simulink model "ALL_JP360_DBW_V6_5_1103"  (R2022a)
settings: Solver=FixedStepAuto  StartTime=0.0  StopTime=inf  FixedStep=0.01  RelTol=1e-3  EnableMultiTasking=on
model workspace (MAT data in the model file):
  g = 9.8
undefined symbols (not defined in the file or in its folder): canChannel, delta_v_p, IPM_Line_C0, IPM_Line_C1, IPM_Line_C2, IPM_Line_C3, M, M_p, MRR_ObjDistX, MRR_ObjDistY, MRR_ObjFusionCamID, MRR_ObjFusionSig, MRR_ObjID, MRR_ObjRelVelX, MRR_ObjRelVelY, MRR_ObjType, MRR_ObjUpdFlg, none, obj_vaild, untracktime, V, videoinput
libraries: canfdmsglib x230, canfdlib x76, slpidlib x24, simulink x18, dspstat3 x14, ctrlSharedLib x1, simulink_extras x1, imaqlib x1, realtime_pacer_lib x1, dspvision x1, visionsinks x1
(part 6 of 55)

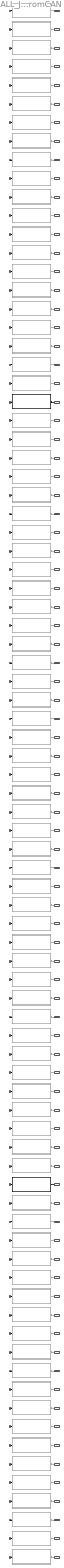
== system ALL_JP360_DBW_V6_5_1103/MsgFromCAN/SRR_ADCU_MsgFromCAN ==
  SRR_ADCU_FLR_AssistSysSt_0x71FromInData : Inport  OutDataTypeStr=Bus:CAN_FD_MESSAGE_BUS
  SRR_ADCU_FLR_Freespace_0x1E1FromInData : Inport  Port=2  OutDataTypeStr=Bus:CAN_FD_MESSAGE_BUS
  SRR_ADCU_FLR_Freespace_0x1E2FromInData : Inport  Port=3  OutDataTypeStr=Bus:CAN_FD_MESSAGE_BUS
  SRR_ADCU_FLR_Freespace_0x1E3FromInData : Inport  Port=4  OutDataTypeStr=Bus:CAN_FD_MESSAGE_BUS
  SRR_ADCU_FLR_Freespace_0x1E4FromInData : Inport  Port=5  OutDataTypeStr=Bus:CAN_FD_MESSAGE_BUS
  SRR_ADCU_FLR_OBJPos10_0x19AFromInData : Inport  Port=6  OutDataTypeStr=Bus:CAN_FD_MESSAGE_BUS
  SRR_ADCU_FLR_OBJPos11_0x19BFromInData : Inport  Port=7  OutDataTypeStr=Bus:CAN_FD_MESSAGE_BUS
  SRR_ADCU_FLR_OBJPos12_0x19CFromInData : Inport  Port=8  OutDataTypeStr=Bus:CAN_FD_MESSAGE_BUS
  SRR_ADCU_FLR_OBJPos13_0x19DFromInData : Inport  Port=9  OutDataTypeStr=Bus:CAN_FD_MESSAGE_BUS
  SRR_ADCU_FLR_OBJPos14_0x19EFromInData : Inport  Port=10  OutDataTypeStr=Bus:CAN_FD_MESSAGE_BUS
  SRR_ADCU_FLR_OBJPos15_0x1A1FromInData : Inport  Port=11  OutDataTypeStr=Bus:CAN_FD_MESSAGE_BUS
  SRR_ADCU_FLR_OBJPos16_0x1A2FromInData : Inport  Port=12  OutDataTypeStr=Bus:CAN_FD_MESSAGE_BUS
  SRR_ADCU_FLR_OBJPos1_0x191FromInData : Inport  Port=13  OutDataTypeStr=Bus:CAN_FD_MESSAGE_BUS
  SRR_ADCU_FLR_OBJPos2_0x192FromInData : Inport  Port=14  OutDataTypeStr=Bus:CAN_FD_MESSAGE_BUS
  SRR_ADCU_FLR_OBJPos3_0x193FromInData : Inport  Port=15  OutDataTypeStr=Bus:CAN_FD_MESSAGE_BUS
  SRR_ADCU_FLR_OBJPos4_0x194FromInData : Inport  Port=16  OutDataTypeStr=Bus:CAN_FD_MESSAGE_BUS
  SRR_ADCU_FLR_OBJPos5_0x195FromInData : Inport  Port=17  OutDataTypeStr=Bus:CAN_FD_MESSAGE_BUS
  SRR_ADCU_FLR_OBJPos6_0x196FromInData : Inport  Port=18  OutDataTypeStr=Bus:CAN_FD_MESSAGE_BUS
  SRR_ADCU_FLR_OBJPos7_0x197FromInData : Inport  Port=19  OutDataTypeStr=Bus:CAN_FD_MESSAGE_BUS
  SRR_ADCU_FLR_OBJPos8_0x198FromInData : Inport  Port=20  OutDataTypeStr=Bus:CAN_FD_MESSAGE_BUS
  SRR_ADCU_FLR_OBJPos9_0x199FromInData : Inport  Port=21  OutDataTypeStr=Bus:CAN_FD_MESSAGE_BUS
  SRR_ADCU_FRR_AssistSysSt_0x72FromInData : Inport  Port=22  OutDataTypeStr=Bus:CAN_FD_MESSAGE_BUS
  SRR_ADCU_FRR_Freespace_1E6FromInData : Inport  Port=23  OutDataTypeStr=Bus:CAN_FD_MESSAGE_BUS
  SRR_ADCU_FRR_Freespace_1E7FromInData : Inport  Port=24  OutDataTypeStr=Bus:CAN_FD_MESSAGE_BUS
  SRR_ADCU_FRR_Freespace_1E8FromInData : Inport  Port=25  OutDataTypeStr=Bus:CAN_FD_MESSAGE_BUS
  SRR_ADCU_FRR_Freespace_1E9FromInData : Inport  Port=26  OutDataTypeStr=Bus:CAN_FD_MESSAGE_BUS
  SRR_ADCU_FRR_OBJPos10_0x1ACFromInData : Inport  Port=27  OutDataTypeStr=Bus:CAN_FD_MESSAGE_BUS
  SRR_ADCU_FRR_OBJPos11_0x1ADFromInData : Inport  Port=28  OutDataTypeStr=Bus:CAN_FD_MESSAGE_BUS
  SRR_ADCU_FRR_OBJPos12_0x1AEFromInData : Inport  Port=29  OutDataTypeStr=Bus:CAN_FD_MESSAGE_BUS
  SRR_ADCU_FRR_OBJPos13_0x1B0FromInData : Inport  Port=30  OutDataTypeStr=Bus:CAN_FD_MESSAGE_BUS
  SRR_ADCU_FRR_OBJPos14_0x1B1FromInData : Inport  Port=31  OutDataTypeStr=Bus:CAN_FD_MESSAGE_BUS
  SRR_ADCU_FRR_OBJPos15_0x1B2FromInData : Inport  Port=32  OutDataTypeStr=Bus:CAN_FD_MESSAGE_BUS
  SRR_ADCU_FRR_OBJPos16_0x1B3FromInData : Inport  Port=33  OutDataTypeStr=Bus:CAN_FD_MESSAGE_BUS
  SRR_ADCU_FRR_OBJPos1_0x1A3FromInData : Inport  Port=34  OutDataTypeStr=Bus:CAN_FD_MESSAGE_BUS
  SRR_ADCU_FRR_OBJPos2_0x1A4FromInData : Inport  Port=35  OutDataTypeStr=Bus:CAN_FD_MESSAGE_BUS
  SRR_ADCU_FRR_OBJPos3_0x1A5FromInData : Inport  Port=36  OutDataTypeStr=Bus:CAN_FD_MESSAGE_BUS
  SRR_ADCU_FRR_OBJPos4_0x1A6FromInData : Inport  Port=37  OutDataTypeStr=Bus:CAN_FD_MESSAGE_BUS
  SRR_ADCU_FRR_OBJPos5_0x1A7FromInData : Inport  Port=38  OutDataTypeStr=Bus:CAN_FD_MESSAGE_BUS
  SRR_ADCU_FRR_OBJPos6_0x1A8FromInData : Inport  Port=39  OutDataTypeStr=Bus:CAN_FD_MESSAGE_BUS
  SRR_ADCU_FRR_OBJPos7_0x1A9FromInData : Inport  Port=40  OutDataTypeStr=Bus:CAN_FD_MESSAGE_BUS
  SRR_ADCU_FRR_OBJPos8_0x1AAFromInData : Inport  Port=41  OutDataTypeStr=Bus:CAN_FD_MESSAGE_BUS
  SRR_ADCU_FRR_OBJPos9_0x1ABFromInData : Inport  Port=42  OutDataTypeStr=Bus:CAN_FD_MESSAGE_BUS
  SRR_ADCU_RLR_AssistSysSt_0x74FromInData : Inport  Port=43  OutDataTypeStr=Bus:CAN_FD_MESSAGE_BUS
  SRR_ADCU_RLR_Freespace_0x1F1FromInData : Inport  Port=44  OutDataTypeStr=Bus:CAN_FD_MESSAGE_BUS
  SRR_ADCU_RLR_Freespace_0x1F2FromInData : Inport  Port=45  OutDataTypeStr=Bus:CAN_FD_MESSAGE_BUS
  SRR_ADCU_RLR_Freespace_0x1F3FromInData : Inport  Port=46  OutDataTypeStr=Bus:CAN_FD_MESSAGE_BUS
  SRR_ADCU_RLR_Freespace_0x1F4FromInData : Inport  Port=47  OutDataTypeStr=Bus:CAN_FD_MESSAGE_BUS
  SRR_ADCU_RLR_OBJPos10_0x1CDFromInData : Inport  Port=48  OutDataTypeStr=Bus:CAN_FD_MESSAGE_BUS
  SRR_ADCU_RLR_OBJPos11_0x1CEFromInData : Inport  Port=49  OutDataTypeStr=Bus:CAN_FD_MESSAGE_BUS
  SRR_ADCU_RLR_OBJPos12_0x1D1FromInData : Inport  Port=50  OutDataTypeStr=Bus:CAN_FD_MESSAGE_BUS
  SRR_ADCU_RLR_OBJPos13_0x1D2FromInData : Inport  Port=51  OutDataTypeStr=Bus:CAN_FD_MESSAGE_BUS
  SRR_ADCU_RLR_OBJPos14_0x1D3FromInData : Inport  Port=52  OutDataTypeStr=Bus:CAN_FD_MESSAGE_BUS
  SRR_ADCU_RLR_OBJPos15_0x1D4FromInData : Inport  Port=53  OutDataTypeStr=Bus:CAN_FD_MESSAGE_BUS
  SRR_ADCU_RLR_OBJPos16_0x1D5FromInData : Inport  Port=54  OutDataTypeStr=Bus:CAN_FD_MESSAGE_BUS
  SRR_ADCU_RLR_OBJPos1_0x1C4FromInData : Inport  Port=55  OutDataTypeStr=Bus:CAN_FD_MESSAGE_BUS
  SRR_ADCU_RLR_OBJPos2_0x1C5FromInData : Inport  Port=56  OutDataTypeStr=Bus:CAN_FD_MESSAGE_BUS
  SRR_ADCU_RLR_OBJPos3_0x1C6FromInData : Inport  Port=57  OutDataTypeStr=Bus:CAN_FD_MESSAGE_BUS
  SRR_ADCU_RLR_OBJPos4_0x1C7FromInData : Inport  Port=58  OutDataTypeStr=Bus:CAN_FD_MESSAGE_BUS
  SRR_ADCU_RLR_OBJPos5_0x1C8FromInData : Inport  Port=59  OutDataTypeStr=Bus:CAN_FD_MESSAGE_BUS
  SRR_ADCU_RLR_OBJPos6_0x1C9FromInData : Inport  Port=60  OutDataTypeStr=Bus:CAN_FD_MESSAGE_BUS
  SRR_ADCU_RLR_OBJPos7_0x1CAFromInData : Inport  Port=61  OutDataTypeStr=Bus:CAN_FD_MESSAGE_BUS
  SRR_ADCU_RLR_OBJPos8_0x1CBFromInData : Inport  Port=62  OutDataTypeStr=Bus:CAN_FD_MESSAGE_BUS
  SRR_ADCU_RLR_OBJPos9_0x1CCFromInData : Inport  Port=63  OutDataTypeStr=Bus:CAN_FD_MESSAGE_BUS
  SRR_ADCU_RRR_AssistSysSt_0x73FromInData : Inport  Port=64  OutDataTypeStr=Bus:CAN_FD_MESSAGE_BUS
  SRR_ADCU_RRR_Freespace_0x1EBFromInData : Inport  Port=65  OutDataTypeStr=Bus:CAN_FD_MESSAGE_BUS
  SRR_ADCU_RRR_Freespace_0x1ECFromInData : Inport  Port=66  OutDataTypeStr=Bus:CAN_FD_MESSAGE_BUS
  SRR_ADCU_RRR_Freespace_0x1EDFromInData : Inport  Port=67  OutDataTypeStr=Bus:CAN_FD_MESSAGE_BUS
  SRR_ADCU_RRR_Freespace_0x1EEFromInData : Inport  Port=68  OutDataTypeStr=Bus:CAN_FD_MESSAGE_BUS
  SRR_ADCU_RRR_OBJPos10_0x1BDFromInData : Inport  Port=69  OutDataTypeStr=Bus:CAN_FD_MESSAGE_BUS
  SRR_ADCU_RRR_OBJPos11_0x1BEFromInData : Inport  Port=70  OutDataTypeStr=Bus:CAN_FD_MESSAGE_BUS
  SRR_ADCU_RRR_OBJPos12_0x1BFFromInData : Inport  Port=71  OutDataTypeStr=Bus:CAN_FD_MESSAGE_BUS
  SRR_ADCU_RRR_OBJPos13_0x1C0FromInData : Inport  Port=72  OutDataTypeStr=Bus:CAN_FD_MESSAGE_BUS
  SRR_ADCU_RRR_OBJPos14_0x1C1FromInData : Inport  Port=73  OutDataTypeStr=Bus:CAN_FD_MESSAGE_BUS
  SRR_ADCU_RRR_OBJPos15_0x1C2FromInData : Inport  Port=74  OutDataTypeStr=Bus:CAN_FD_MESSAGE_BUS
  SRR_ADCU_RRR_OBJPos16_0x1C3FromInData : Inport  Port=75  OutDataTypeStr=Bus:CAN_FD_MESSAGE_BUS
  SRR_ADCU_RRR_OBJPos1_0x1B4FromInData : Inport  Port=76  OutDataTypeStr=Bus:CAN_FD_MESSAGE_BUS
  SRR_ADCU_RRR_OBJPos2_0x1B5FromInData : Inport  Port=77  OutDataTypeStr=Bus:CAN_FD_MESSAGE_BUS
  SRR_ADCU_RRR_OBJPos3_0x1B6FromInData : Inport  Port=78  OutDataTypeStr=Bus:CAN_FD_MESSAGE_BUS
  SRR_ADCU_RRR_OBJPos4_0x1B7FromInData : Inport  Port=79  OutDataTypeStr=Bus:CAN_FD_MESSAGE_BUS
  SRR_ADCU_RRR_OBJPos5_0x1B8FromInData : Inport  Port=80  OutDataTypeStr=Bus:CAN_FD_MESSAGE_BUS
  SRR_ADCU_RRR_OBJPos6_0x1B9FromInData : Inport  Port=81  OutDataTypeStr=Bus:CAN_FD_MESSAGE_BUS
  SRR_ADCU_RRR_OBJPos7_0x1BAFromInData : Inport  Port=82  OutDataTypeStr=Bus:CAN_FD_MESSAGE_BUS
  SRR_ADCU_RRR_OBJPos8_0x1BBFromInData : Inport  Port=83  OutDataTypeStr=Bus:CAN_FD_MESSAGE_BUS
  SRR_ADCU_RRR_OBJPos9_0x1BCFromInData : Inport  Port=84  OutDataTypeStr=Bus:CAN_FD_MESSAGE_BUS
  SRR_ADCU_FLR_AssistSysSt_0x71 : Subsystem  Commented=on  TreatAsAtomicUnit=on
  SRR_ADCU_FLR_Freespace_0x1E1 : Subsystem  Commented=on  TreatAsAtomicUnit=on
  SRR_ADCU_FLR_Freespace_0x1E2 : Subsystem  Commented=on  TreatAsAtomicUnit=on
  SRR_ADCU_FLR_Freespace_0x1E3 : Subsystem  Commented=on  TreatAsAtomicUnit=on
  SRR_ADCU_FLR_Freespace_0x1E4 : Subsystem  Commented=on  TreatAsAtomicUnit=on
  SRR_ADCU_FLR_OBJPos10_0x19A : Subsystem  Commented=on  TreatAsAtomicUnit=on
  SRR_ADCU_FLR_OBJPos11_0x19B : Subsystem  Commented=on  TreatAsAtomicUnit=on
  SRR_ADCU_FLR_OBJPos12_0x19C : Subsystem  Commented=on  TreatAsAtomicUnit=on
  SRR_ADCU_FLR_OBJPos13_0x19D : Subsystem  Commented=on  TreatAsAtomicUnit=on
  SRR_ADCU_FLR_OBJPos14_0x19E : Subsystem  Commented=on  TreatAsAtomicUnit=on
  SRR_ADCU_FLR_OBJPos15_0x1A1 : Subsystem  Commented=on  TreatAsAtomicUnit=on
  SRR_ADCU_FLR_OBJPos16_0x1A2 : Subsystem  Commented=on  TreatAsAtomicUnit=on
  SRR_ADCU_FLR_OBJPos1_0x191 : Subsystem  Commented=on  TreatAsAtomicUnit=on
  SRR_ADCU_FLR_OBJPos2_0x192 : Subsystem  Commented=on  TreatAsAtomicUnit=on
  SRR_ADCU_FLR_OBJPos3_0x193 : Subsystem  Commented=on  TreatAsAtomicUnit=on
  SRR_ADCU_FLR_OBJPos4_0x194 : Subsystem  Commented=on  TreatAsAtomicUnit=on
  SRR_ADCU_FLR_OBJPos5_0x195 : Subsystem  Commented=on  TreatAsAtomicUnit=on
  SRR_ADCU_FLR_OBJPos6_0x196 : Subsystem  Commented=on  TreatAsAtomicUnit=on
  SRR_ADCU_FLR_OBJPos7_0x197 : Subsystem  Commented=on  TreatAsAtomicUnit=on
  SRR_ADCU_FLR_OBJPos8_0x198 : Subsystem  Commented=on  TreatAsAtomicUnit=on
  SRR_ADCU_FLR_OBJPos9_0x199 : Subsystem  Commented=on  TreatAsAtomicUnit=on
  SRR_ADCU_FRR_AssistSysSt_0x72 : Subsystem  TreatAsAtomicUnit=on
  SRR_ADCU_FRR_Freespace_1E6 : Subsystem  Commented=on  TreatAsAtomicUnit=on
  SRR_ADCU_FRR_Freespace_1E7 : Subsystem  Commented=on  TreatAsAtomicUnit=on
  SRR_ADCU_FRR_Freespace_1E8 : Subsystem  Commented=on  TreatAsAtomicUnit=on
  SRR_ADCU_FRR_Freespace_1E9 : Subsystem  Commented=on  TreatAsAtomicUnit=on
  SRR_ADCU_FRR_OBJPos10_0x1AC : Subsystem  Commented=on  TreatAsAtomicUnit=on
  SRR_ADCU_FRR_OBJPos11_0x1AD : Subsystem  Commented=on  TreatAsAtomicUnit=on
  SRR_ADCU_FRR_OBJPos12_0x1AE : Subsystem  Commented=on  TreatAsAtomicUnit=on
  SRR_ADCU_FRR_OBJPos13_0x1B0 : Subsystem  Commented=on  TreatAsAtomicUnit=on
  SRR_ADCU_FRR_OBJPos14_0x1B1 : Subsystem  Commented=on  TreatAsAtomicUnit=on
  SRR_ADCU_FRR_OBJPos15_0x1B2 : Subsystem  Commented=on  TreatAsAtomicUnit=on
  SRR_ADCU_FRR_OBJPos16_0x1B3 : Subsystem  Commented=on  TreatAsAtomicUnit=on
  SRR_ADCU_FRR_OBJPos1_0x1A3 : Subsystem  Commented=on  TreatAsAtomicUnit=on
  SRR_ADCU_FRR_OBJPos2_0x1A4 : Subsystem  Commented=on  TreatAsAtomicUnit=on
  SRR_ADCU_FRR_OBJPos3_0x1A5 : Subsystem  Commented=on  TreatAsAtomicUnit=on
  SRR_ADCU_FRR_OBJPos4_0x1A6 : Subsystem  Commented=on  TreatAsAtomicUnit=on
  SRR_ADCU_FRR_OBJPos5_0x1A7 : Subsystem  Commented=on  TreatAsAtomicUnit=on
  SRR_ADCU_FRR_OBJPos6_0x1A8 : Subsystem  Commented=on  TreatAsAtomicUnit=on
  SRR_ADCU_FRR_OBJPos7_0x1A9 : Subsystem  Commented=on  TreatAsAtomicUnit=on
  SRR_ADCU_FRR_OBJPos8_0x1AA : Subsystem  Commented=on  TreatAsAtomicUnit=on
  SRR_ADCU_FRR_OBJPos9_0x1AB : Subsystem  Commented=on  TreatAsAtomicUnit=on
  SRR_ADCU_RLR_AssistSysSt_0x74 : Subsystem  Commented=on  TreatAsAtomicUnit=on
  SRR_ADCU_RLR_Freespace_0x1F1 : Subsystem  Commented=on  TreatAsAtomicUnit=on
  SRR_ADCU_RLR_Freespace_0x1F2 : Subsystem  Commented=on  TreatAsAtomicUnit=on
  SRR_ADCU_RLR_Freespace_0x1F3 : Subsystem  Commented=on  TreatAsAtomicUnit=on
  SRR_ADCU_RLR_Freespace_0x1F4 : Subsystem  Commented=on  TreatAsAtomicUnit=on
  SRR_ADCU_RLR_OBJPos10_0x1CD : Subsystem  Commented=on  TreatAsAtomicUnit=on
  SRR_ADCU_RLR_OBJPos11_0x1CE : Subsystem  Commented=on  TreatAsAtomicUnit=on
  SRR_ADCU_RLR_OBJPos12_0x1D1 : Subsystem  Commented=on  TreatAsAtomicUnit=on
  SRR_ADCU_RLR_OBJPos13_0x1D2 : Subsystem  Commented=on  TreatAsAtomicUnit=on
  SRR_ADCU_RLR_OBJPos14_0x1D3 : Subsystem  Commented=on  TreatAsAtomicUnit=on
  SRR_ADCU_RLR_OBJPos15_0x1D4 : Subsystem  Commented=on  TreatAsAtomicUnit=on
  SRR_ADCU_RLR_OBJPos16_0x1D5 : Subsystem  Commented=on  TreatAsAtomicUnit=on
  SRR_ADCU_RLR_OBJPos1_0x1C4 : Subsystem  Commented=on  TreatAsAtomicUnit=on
  SRR_ADCU_RLR_OBJPos2_0x1C5 : Subsystem  Commented=on  TreatAsAtomicUnit=on
  SRR_ADCU_RLR_OBJPos3_0x1C6 : Subsystem  Commented=on  TreatAsAtomicUnit=on
  SRR_ADCU_RLR_OBJPos4_0x1C7 : Subsystem  Commented=on  TreatAsAtomicUnit=on
  SRR_ADCU_RLR_OBJPos5_0x1C8 : Subsystem  Commented=on  TreatAsAtomicUnit=on
  SRR_ADCU_RLR_OBJPos6_0x1C9 : Subsystem  Commented=on  TreatAsAtomicUnit=on
  SRR_ADCU_RLR_OBJPos7_0x1CA : Subsystem  Commented=on  TreatAsAtomicUnit=on
  SRR_ADCU_RLR_OBJPos8_0x1CB : Subsystem  Commented=on  TreatAsAtomicUnit=on
  SRR_ADCU_RLR_OBJPos9_0x1CC : Subsystem  Commented=on  TreatAsAtomicUnit=on
  SRR_ADCU_RRR_AssistSysSt_0x73 : Subsystem  TreatAsAtomicUnit=on
  SRR_ADCU_RRR_Freespace_0x1EB : Subsystem  Commented=on  TreatAsAtomicUnit=on
  SRR_ADCU_RRR_Freespace_0x1EC : Subsystem  Commented=on  TreatAsAtomicUnit=on
  SRR_ADCU_RRR_Freespace_0x1ED : Subsystem  Commented=on  TreatAsAtomicUnit=on
  SRR_ADCU_RRR_Freespace_0x1EE : Subsystem  Commented=on  TreatAsAtomicUnit=on
  SRR_ADCU_RRR_OBJPos10_0x1BD : Subsystem  Commented=on  TreatAsAtomicUnit=on
  SRR_ADCU_RRR_OBJPos11_0x1BE : Subsystem  Commented=on  TreatAsAtomicUnit=on
  SRR_ADCU_RRR_OBJPos12_0x1BF : Subsystem  Commented=on  TreatAsAtomicUnit=on
  SRR_ADCU_RRR_OBJPos13_0x1C0 : Subsystem  Commented=on  TreatAsAtomicUnit=on
  SRR_ADCU_RRR_OBJPos14_0x1C1 : Subsystem  Commented=on  TreatAsAtomicUnit=on
  SRR_ADCU_RRR_OBJPos15_0x1C2 : Subsystem  Commented=on  TreatAsAtomicUnit=on
  SRR_ADCU_RRR_OBJPos16_0x1C3 : Subsystem  Commented=on  TreatAsAtomicUnit=on
  SRR_ADCU_RRR_OBJPos1_0x1B4 : Subsystem  Commented=on  TreatAsAtomicUnit=on
  SRR_ADCU_RRR_OBJPos2_0x1B5 : Subsystem  Commented=on  TreatAsAtomicUnit=on
  SRR_ADCU_RRR_OBJPos3_0x1B6 : Subsystem  Commented=on  TreatAsAtomicUnit=on
  SRR_ADCU_RRR_OBJPos4_0x1B7 : Subsystem  Commented=on  TreatAsAtomicUnit=on
  SRR_ADCU_RRR_OBJPos5_0x1B8 : Subsystem  Commented=on  TreatAsAtomicUnit=on
  SRR_ADCU_RRR_OBJPos6_0x1B9 : Subsystem  Commented=on  TreatAsAtomicUnit=on
  SRR_ADCU_RRR_OBJPos7_0x1BA : Subsystem  Commented=on  TreatAsAtomicUnit=on
  SRR_ADCU_RRR_OBJPos8_0x1BB : Subsystem  Commented=on  TreatAsAtomicUnit=on
  SRR_ADCU_RRR_OBJPos9_0x1BC : Subsystem  Commented=on  TreatAsAtomicUnit=on
  SRR_ADCU_FLR_AssistSysSt_0x71FromOutData : Outport  OutDataTypeStr=Bus:SRR_ADCU_FLR_AssistSysSt_0x71
  SRR_ADCU_FLR_Freespace_0x1E1FromOutData : Outport  Port=2  OutDataTypeStr=Bus:SRR_ADCU_FLR_Freespace_0x1E1
  SRR_ADCU_FLR_Freespace_0x1E2FromOutData : Outport  Port=3  OutDataTypeStr=Bus:SRR_ADCU_FLR_Freespace_0x1E2
  SRR_ADCU_FLR_Freespace_0x1E3FromOutData : Outport  Port=4  OutDataTypeStr=Bus:SRR_ADCU_FLR_Freespace_0x1E3
  SRR_ADCU_FLR_Freespace_0x1E4FromOutData : Outport  Port=5  OutDataTypeStr=Bus:SRR_ADCU_FLR_Freespace_0x1E4
  SRR_ADCU_FLR_OBJPos10_0x19AFromOutData : Outport  Port=6  OutDataTypeStr=Bus:SRR_ADCU_FLR_OBJPos10_0x19A
  SRR_ADCU_FLR_OBJPos11_0x19BFromOutData : Outport  Port=7  OutDataTypeStr=Bus:SRR_ADCU_FLR_OBJPos11_0x19B
  SRR_ADCU_FLR_OBJPos12_0x19CFromOutData : Outport  Port=8  OutDataTypeStr=Bus:SRR_ADCU_FLR_OBJPos12_0x19C
  SRR_ADCU_FLR_OBJPos13_0x19DFromOutData : Outport  Port=9  OutDataTypeStr=Bus:SRR_ADCU_FLR_OBJPos13_0x19D
  SRR_ADCU_FLR_OBJPos14_0x19EFromOutData : Outport  Port=10  OutDataTypeStr=Bus:SRR_ADCU_FLR_OBJPos14_0x19E
  SRR_ADCU_FLR_OBJPos15_0x1A1FromOutData : Outport  Port=11  OutDataTypeStr=Bus:SRR_ADCU_FLR_OBJPos15_0x1A1
  SRR_ADCU_FLR_OBJPos16_0x1A2FromOutData : Outport  Port=12  OutDataTypeStr=Bus:SRR_ADCU_FLR_OBJPos16_0x1A2
  SRR_ADCU_FLR_OBJPos1_0x191FromOutData : Outport  Port=13  OutDataTypeStr=Bus:SRR_ADCU_FLR_OBJPos1_0x191
  SRR_ADCU_FLR_OBJPos2_0x192FromOutData : Outport  Port=14  OutDataTypeStr=Bus:SRR_ADCU_FLR_OBJPos2_0x192
  SRR_ADCU_FLR_OBJPos3_0x193FromOutData : Outport  Port=15  OutDataTypeStr=Bus:SRR_ADCU_FLR_OBJPos3_0x193
  SRR_ADCU_FLR_OBJPos4_0x194FromOutData : Outport  Port=16  OutDataTypeStr=Bus:SRR_ADCU_FLR_OBJPos4_0x194
  SRR_ADCU_FLR_OBJPos5_0x195FromOutData : Outport  Port=17  OutDataTypeStr=Bus:SRR_ADCU_FLR_OBJPos5_0x195
  SRR_ADCU_FLR_OBJPos6_0x196FromOutData : Outport  Port=18  OutDataTypeStr=Bus:SRR_ADCU_FLR_OBJPos6_0x196
  SRR_ADCU_FLR_OBJPos7_0x197FromOutData : Outport  Port=19  OutDataTypeStr=Bus:SRR_ADCU_FLR_OBJPos7_0x197
  SRR_ADCU_FLR_OBJPos8_0x198FromOutData : Outport  Port=20  OutDataTypeStr=Bus:SRR_ADCU_FLR_OBJPos8_0x198
  SRR_ADCU_FLR_OBJPos9_0x199FromOutData : Outport  Port=21  OutDataTypeStr=Bus:SRR_ADCU_FLR_OBJPos9_0x199
  SRR_ADCU_FRR_AssistSysSt_0x72FromOutData : Outport  Port=22  OutDataTypeStr=Bus:SRR_ADCU_FRR_AssistSysSt_0x72
  SRR_ADCU_FRR_Freespace_1E6FromOutData : Outport  Port=23  OutDataTypeStr=Bus:SRR_ADCU_FRR_Freespace_1E6
  SRR_ADCU_FRR_Freespace_1E7FromOutData : Outport  Port=24  OutDataTypeStr=Bus:SRR_ADCU_FRR_Freespace_1E7
  SRR_ADCU_FRR_Freespace_1E8FromOutData : Outport  Port=25  OutDataTypeStr=Bus:SRR_ADCU_FRR_Freespace_1E8
  SRR_ADCU_FRR_Freespace_1E9FromOutData : Outport  Port=26  OutDataTypeStr=Bus:SRR_ADCU_FRR_Freespace_1E9
  SRR_ADCU_FRR_OBJPos10_0x1ACFromOutData : Outport  Port=27  OutDataTypeStr=Bus:SRR_ADCU_FRR_OBJPos10_0x1AC
  SRR_ADCU_FRR_OBJPos11_0x1ADFromOutData : Outport  Port=28  OutDataTypeStr=Bus:SRR_ADCU_FRR_OBJPos11_0x1AD
  SRR_ADCU_FRR_OBJPos12_0x1AEFromOutData : Outport  Port=29  OutDataTypeStr=Bus:SRR_ADCU_FRR_OBJPos12_0x1AE
  SRR_ADCU_FRR_OBJPos13_0x1B0FromOutData : Outport  Port=30  OutDataTypeStr=Bus:SRR_ADCU_FRR_OBJPos13_0x1B0
  SRR_ADCU_FRR_OBJPos14_0x1B1FromOutData : Outport  Port=31  OutDataTypeStr=Bus:SRR_ADCU_FRR_OBJPos14_0x1B1
  SRR_ADCU_FRR_OBJPos15_0x1B2FromOutData : Outport  Port=32  OutDataTypeStr=Bus:SRR_ADCU_FRR_OBJPos15_0x1B2
  SRR_ADCU_FRR_OBJPos16_0x1B3FromOutData : Outport  Port=33  OutDataTypeStr=Bus:SRR_ADCU_FRR_OBJPos16_0x1B3
  SRR_ADCU_FRR_OBJPos1_0x1A3FromOutData : Outport  Port=34  OutDataTypeStr=Bus:SRR_ADCU_FRR_OBJPos1_0x1A3
  SRR_ADCU_FRR_OBJPos2_0x1A4FromOutData : Outport  Port=35  OutDataTypeStr=Bus:SRR_ADCU_FRR_OBJPos2_0x1A4
  SRR_ADCU_FRR_OBJPos3_0x1A5FromOutData : Outport  Port=36  OutDataTypeStr=Bus:SRR_ADCU_FRR_OBJPos3_0x1A5
  SRR_ADCU_FRR_OBJPos4_0x1A6FromOutData : Outport  Port=37  OutDataTypeStr=Bus:SRR_ADCU_FRR_OBJPos4_0x1A6
  SRR_ADCU_FRR_OBJPos5_0x1A7FromOutData : Outport  Port=38  OutDataTypeStr=Bus:SRR_ADCU_FRR_OBJPos5_0x1A7
  SRR_ADCU_FRR_OBJPos6_0x1A8FromOutData : Outport  Port=39  OutDataTypeStr=Bus:SRR_ADCU_FRR_OBJPos6_0x1A8
  SRR_ADCU_FRR_OBJPos7_0x1A9FromOutData : Outport  Port=40  OutDataTypeStr=Bus:SRR_ADCU_FRR_OBJPos7_0x1A9
  SRR_ADCU_FRR_OBJPos8_0x1AAFromOutData : Outport  Port=41  OutDataTypeStr=Bus:SRR_ADCU_FRR_OBJPos8_0x1AA
  SRR_ADCU_FRR_OBJPos9_0x1ABFromOutData : Outport  Port=42  OutDataTypeStr=Bus:SRR_ADCU_FRR_OBJPos9_0x1AB
  SRR_ADCU_RLR_AssistSysSt_0x74FromOutData : Outport  Port=43  OutDataTypeStr=Bus:SRR_ADCU_RLR_AssistSysSt_0x74
  SRR_ADCU_RLR_Freespace_0x1F1FromOutData : Outport  Port=44  OutDataTypeStr=Bus:SRR_ADCU_RLR_Freespace_0x1F1
  SRR_ADCU_RLR_Freespace_0x1F2FromOutData : Outport  Port=45  OutDataTypeStr=Bus:SRR_ADCU_RLR_Freespace_0x1F2
  SRR_ADCU_RLR_Freespace_0x1F3FromOutData : Outport  Port=46  OutDataTypeStr=Bus:SRR_ADCU_RLR_Freespace_0x1F3
  SRR_ADCU_RLR_Freespace_0x1F4FromOutData : Outport  Port=47  OutDataTypeStr=Bus:SRR_ADCU_RLR_Freespace_0x1F4
  SRR_ADCU_RLR_OBJPos10_0x1CDFromOutData : Outport  Port=48  OutDataTypeStr=Bus:SRR_ADCU_RLR_OBJPos10_0x1CD
  SRR_ADCU_RLR_OBJPos11_0x1CEFromOutData : Outport  Port=49  OutDataTypeStr=Bus:SRR_ADCU_RLR_OBJPos11_0x1CE
  SRR_ADCU_RLR_OBJPos12_0x1D1FromOutData : Outport  Port=50  OutDataTypeStr=Bus:SRR_ADCU_RLR_OBJPos12_0x1D1
  SRR_ADCU_RLR_OBJPos13_0x1D2FromOutData : Outport  Port=51  OutDataTypeStr=Bus:SRR_ADCU_RLR_OBJPos13_0x1D2
  SRR_ADCU_RLR_OBJPos14_0x1D3FromOutData : Outport  Port=52  OutDataTypeStr=Bus:SRR_ADCU_RLR_OBJPos14_0x1D3
  SRR_ADCU_RLR_OBJPos15_0x1D4FromOutData : Outport  Port=53  OutDataTypeStr=Bus:SRR_ADCU_RLR_OBJPos15_0x1D4
  SRR_ADCU_RLR_OBJPos16_0x1D5FromOutData : Outport  Port=54  OutDataTypeStr=Bus:SRR_ADCU_RLR_OBJPos16_0x1D5
  SRR_ADCU_RLR_OBJPos1_0x1C4FromOutData : Outport  Port=55  OutDataTypeStr=Bus:SRR_ADCU_RLR_OBJPos1_0x1C4
  SRR_ADCU_RLR_OBJPos2_0x1C5FromOutData : Outport  Port=56  OutDataTypeStr=Bus:SRR_ADCU_RLR_OBJPos2_0x1C5
  SRR_ADCU_RLR_OBJPos3_0x1C6FromOutData : Outport  Port=57  OutDataTypeStr=Bus:SRR_ADCU_RLR_OBJPos3_0x1C6
  SRR_ADCU_RLR_OBJPos4_0x1C7FromOutData : Outport  Port=58  OutDataTypeStr=Bus:SRR_ADCU_RLR_OBJPos4_0x1C7
  SRR_ADCU_RLR_OBJPos5_0x1C8FromOutData : Outport  Port=59  OutDataTypeStr=Bus:SRR_ADCU_RLR_OBJPos5_0x1C8
  SRR_ADCU_RLR_OBJPos6_0x1C9FromOutData : Outport  Port=60  OutDataTypeStr=Bus:SRR_ADCU_RLR_OBJPos6_0x1C9
  SRR_ADCU_RLR_OBJPos7_0x1CAFromOutData : Outport  Port=61  OutDataTypeStr=Bus:SRR_ADCU_RLR_OBJPos7_0x1CA
  SRR_ADCU_RLR_OBJPos8_0x1CBFromOutData : Outport  Port=62  OutDataTypeStr=Bus:SRR_ADCU_RLR_OBJPos8_0x1CB
  SRR_ADCU_RLR_OBJPos9_0x1CCFromOutData : Outport  Port=63  OutDataTypeStr=Bus:SRR_ADCU_RLR_OBJPos9_0x1CC
  SRR_ADCU_RRR_AssistSysSt_0x73FromOutData : Outport  Port=64  OutDataTypeStr=Bus:SRR_ADCU_RRR_AssistSysSt_0x73
  SRR_ADCU_RRR_Freespace_0x1EBFromOutData : Outport  Port=65  OutDataTypeStr=Bus:SRR_ADCU_RRR_Freespace_0x1EB
  SRR_ADCU_RRR_Freespace_0x1ECFromOutData : Outport  Port=66  OutDataTypeStr=Bus:SRR_ADCU_RRR_Freespace_0x1EC
  SRR_ADCU_RRR_Freespace_0x1EDFromOutData : Outport  Port=67  OutDataTypeStr=Bus:SRR_ADCU_RRR_Freespace_0x1ED
  SRR_ADCU_RRR_Freespace_0x1EEFromOutData : Outport  Port=68  OutDataTypeStr=Bus:SRR_ADCU_RRR_Freespace_0x1EE
  SRR_ADCU_RRR_OBJPos10_0x1BDFromOutData : Outport  Port=69  OutDataTypeStr=Bus:SRR_ADCU_RRR_OBJPos10_0x1BD
  SRR_ADCU_RRR_OBJPos11_0x1BEFromOutData : Outport  Port=70  OutDataTypeStr=Bus:SRR_ADCU_RRR_OBJPos11_0x1BE
  SRR_ADCU_RRR_OBJPos12_0x1BFFromOutData : Outport  Port=71  OutDataTypeStr=Bus:SRR_ADCU_RRR_OBJPos12_0x1BF
  SRR_ADCU_RRR_OBJPos13_0x1C0FromOutData : Outport  Port=72  OutDataTypeStr=Bus:SRR_ADCU_RRR_OBJPos13_0x1C0
  SRR_ADCU_RRR_OBJPos14_0x1C1FromOutData : Outport  Port=73  OutDataTypeStr=Bus:SRR_ADCU_RRR_OBJPos14_0x1C1
  SRR_ADCU_RRR_OBJPos15_0x1C2FromOutData : Outport  Port=74  OutDataTypeStr=Bus:SRR_ADCU_RRR_OBJPos15_0x1C2
  SRR_ADCU_RRR_OBJPos16_0x1C3FromOutData : Outport  Port=75  OutDataTypeStr=Bus:SRR_ADCU_RRR_OBJPos16_0x1C3
  SRR_ADCU_RRR_OBJPos1_0x1B4FromOutData : Outport  Port=76  OutDataTypeStr=Bus:SRR_ADCU_RRR_OBJPos1_0x1B4
  SRR_ADCU_RRR_OBJPos2_0x1B5FromOutData : Outport  Port=77  OutDataTypeStr=Bus:SRR_ADCU_RRR_OBJPos2_0x1B5
  SRR_ADCU_RRR_OBJPos3_0x1B6FromOutData : Outport  Port=78  OutDataTypeStr=Bus:SRR_ADCU_RRR_OBJPos3_0x1B6
  SRR_ADCU_RRR_OBJPos4_0x1B7FromOutData : Outport  Port=79  OutDataTypeStr=Bus:SRR_ADCU_RRR_OBJPos4_0x1B7
  SRR_ADCU_RRR_OBJPos5_0x1B8FromOutData : Outport  Port=80  OutDataTypeStr=Bus:SRR_ADCU_RRR_OBJPos5_0x1B8
  SRR_ADCU_RRR_OBJPos6_0x1B9FromOutData : Outport  Port=81  OutDataTypeStr=Bus:SRR_ADCU_RRR_OBJPos6_0x1B9
  SRR_ADCU_RRR_OBJPos7_0x1BAFromOutData : Outport  Port=82  OutDataTypeStr=Bus:SRR_ADCU_RRR_OBJPos7_0x1BA
  SRR_ADCU_RRR_OBJPos8_0x1BBFromOutData : Outport  Port=83  OutDataTypeStr=Bus:SRR_ADCU_RRR_OBJPos8_0x1BB
  SRR_ADCU_RRR_OBJPos9_0x1BCFromOutData : Outport  Port=84  OutDataTypeStr=Bus:SRR_ADCU_RRR_OBJPos9_0x1BC
  wires:
  SRR_ADCU_FLR_AssistSysSt_0x71/1(SRR_ADCU_FLR_AssistSysSt_0x71FromOutData) -> SRR_ADCU_FLR_AssistSysSt_0x71FromOutData/1  "SRR_ADCU_FLR_AssistSysSt_0x71FromOutData"
  SRR_ADCU_FLR_AssistSysSt_0x71FromInData/1 -> SRR_ADCU_FLR_AssistSysSt_0x71/1(SRR_ADCU_FLR_AssistSysSt_0x71FromInData)  "SRR_ADCU_FLR_AssistSysSt_0x71FromInData"
  SRR_ADCU_FLR_Freespace_0x1E1/1(SRR_ADCU_FLR_Freespace_0x1E1FromOutData) -> SRR_ADCU_FLR_Freespace_0x1E1FromOutData/1  "SRR_ADCU_FLR_Freespace_0x1E1FromOutData"
  SRR_ADCU_FLR_Freespace_0x1E1FromInData/1 -> SRR_ADCU_FLR_Freespace_0x1E1/1(SRR_ADCU_FLR_Freespace_0x1E1FromInData)  "SRR_ADCU_FLR_Freespace_0x1E1FromInData"
  SRR_ADCU_FLR_Freespace_0x1E2/1(SRR_ADCU_FLR_Freespace_0x1E2FromOutData) -> SRR_ADCU_FLR_Freespace_0x1E2FromOutData/1  "SRR_ADCU_FLR_Freespace_0x1E2FromOutData"
  SRR_ADCU_FLR_Freespace_0x1E2FromInData/1 -> SRR_ADCU_FLR_Freespace_0x1E2/1(SRR_ADCU_FLR_Freespace_0x1E2FromInData)  "SRR_ADCU_FLR_Freespace_0x1E2FromInData"
  SRR_ADCU_FLR_Freespace_0x1E3/1(SRR_ADCU_FLR_Freespace_0x1E3FromOutData) -> SRR_ADCU_FLR_Freespace_0x1E3FromOutData/1  "SRR_ADCU_FLR_Freespace_0x1E3FromOutData"
  SRR_ADCU_FLR_Freespace_0x1E3FromInData/1 -> SRR_ADCU_FLR_Freespace_0x1E3/1(SRR_ADCU_FLR_Freespace_0x1E3FromInData)  "SRR_ADCU_FLR_Freespace_0x1E3FromInData"
  SRR_ADCU_FLR_Freespace_0x1E4/1(SRR_ADCU_FLR_Freespace_0x1E4FromOutData) -> SRR_ADCU_FLR_Freespace_0x1E4FromOutData/1  "SRR_ADCU_FLR_Freespace_0x1E4FromOutData"
  SRR_ADCU_FLR_Freespace_0x1E4FromInData/1 -> SRR_ADCU_FLR_Freespace_0x1E4/1(SRR_ADCU_FLR_Freespace_0x1E4FromInData)  "SRR_ADCU_FLR_Freespace_0x1E4FromInData"
  SRR_ADCU_FLR_OBJPos10_0x19A/1(SRR_ADCU_FLR_OBJPos10_0x19AFromOutData) -> SRR_ADCU_FLR_OBJPos10_0x19AFromOutData/1  "SRR_ADCU_FLR_OBJPos10_0x19AFromOutData"
  SRR_ADCU_FLR_OBJPos10_0x19AFromInData/1 -> SRR_ADCU_FLR_OBJPos10_0x19A/1(SRR_ADCU_FLR_OBJPos10_0x19AFromInData)  "SRR_ADCU_FLR_OBJPos10_0x19AFromInData"
  SRR_ADCU_FLR_OBJPos11_0x19B/1(SRR_ADCU_FLR_OBJPos11_0x19BFromOutData) -> SRR_ADCU_FLR_OBJPos11_0x19BFromOutData/1  "SRR_ADCU_FLR_OBJPos11_0x19BFromOutData"
  SRR_ADCU_FLR_OBJPos11_0x19BFromInData/1 -> SRR_ADCU_FLR_OBJPos11_0x19B/1(SRR_ADCU_FLR_OBJPos11_0x19BFromInData)  "SRR_ADCU_FLR_OBJPos11_0x19BFromInData"
  SRR_ADCU_FLR_OBJPos12_0x19C/1(SRR_ADCU_FLR_OBJPos12_0x19CFromOutData) -> SRR_ADCU_FLR_OBJPos12_0x19CFromOutData/1  "SRR_ADCU_FLR_OBJPos12_0x19CFromOutData"
  SRR_ADCU_FLR_OBJPos12_0x19CFromInData/1 -> SRR_ADCU_FLR_OBJPos12_0x19C/1(SRR_ADCU_FLR_OBJPos12_0x19CFromInData)  "SRR_ADCU_FLR_OBJPos12_0x19CFromInData"
  SRR_ADCU_FLR_OBJPos13_0x19D/1(SRR_ADCU_FLR_OBJPos13_0x19DFromOutData) -> SRR_ADCU_FLR_OBJPos13_0x19DFromOutData/1  "SRR_ADCU_FLR_OBJPos13_0x19DFromOutData"
  SRR_ADCU_FLR_OBJPos13_0x19DFromInData/1 -> SRR_ADCU_FLR_OBJPos13_0x19D/1(SRR_ADCU_FLR_OBJPos13_0x19DFromInData)  "SRR_ADCU_FLR_OBJPos13_0x19DFromInData"
  SRR_ADCU_FLR_OBJPos14_0x19E/1(SRR_ADCU_FLR_OBJPos14_0x19EFromOutData) -> SRR_ADCU_FLR_OBJPos14_0x19EFromOutData/1  "SRR_ADCU_FLR_OBJPos14_0x19EFromOutData"
  SRR_ADCU_FLR_OBJPos14_0x19EFromInData/1 -> SRR_ADCU_FLR_OBJPos14_0x19E/1(SRR_ADCU_FLR_OBJPos14_0x19EFromInData)  "SRR_ADCU_FLR_OBJPos14_0x19EFromInData"
  SRR_ADCU_FLR_OBJPos15_0x1A1/1(SRR_ADCU_FLR_OBJPos15_0x1A1FromOutData) -> SRR_ADCU_FLR_OBJPos15_0x1A1FromOutData/1  "SRR_ADCU_FLR_OBJPos15_0x1A1FromOutData"
  SRR_ADCU_FLR_OBJPos15_0x1A1FromInData/1 -> SRR_ADCU_FLR_OBJPos15_0x1A1/1(SRR_ADCU_FLR_OBJPos15_0x1A1FromInData)  "SRR_ADCU_FLR_OBJPos15_0x1A1FromInData"
  SRR_ADCU_FLR_OBJPos16_0x1A2/1(SRR_ADCU_FLR_OBJPos16_0x1A2FromOutData) -> SRR_ADCU_FLR_OBJPos16_0x1A2FromOutData/1  "SRR_ADCU_FLR_OBJPos16_0x1A2FromOutData"
  SRR_ADCU_FLR_OBJPos16_0x1A2FromInData/1 -> SRR_ADCU_FLR_OBJPos16_0x1A2/1(SRR_ADCU_FLR_OBJPos16_0x1A2FromInData)  "SRR_ADCU_FLR_OBJPos16_0x1A2FromInData"
  SRR_ADCU_FLR_OBJPos1_0x191/1(SRR_ADCU_FLR_OBJPos1_0x191FromOutData) -> SRR_ADCU_FLR_OBJPos1_0x191FromOutData/1  "SRR_ADCU_FLR_OBJPos1_0x191FromOutData"
  SRR_ADCU_FLR_OBJPos1_0x191FromInData/1 -> SRR_ADCU_FLR_OBJPos1_0x191/1(SRR_ADCU_FLR_OBJPos1_0x191FromInData)  "SRR_ADCU_FLR_OBJPos1_0x191FromInData"
  SRR_ADCU_FLR_OBJPos2_0x192/1(SRR_ADCU_FLR_OBJPos2_0x192FromOutData) -> SRR_ADCU_FLR_OBJPos2_0x192FromOutData/1  "SRR_ADCU_FLR_OBJPos2_0x192FromOutData"
  SRR_ADCU_FLR_OBJPos2_0x192FromInData/1 -> SRR_ADCU_FLR_OBJPos2_0x192/1(SRR_ADCU_FLR_OBJPos2_0x192FromInData)  "SRR_ADCU_FLR_OBJPos2_0x192FromInData"
  SRR_ADCU_FLR_OBJPos3_0x193/1(SRR_ADCU_FLR_OBJPos3_0x193FromOutData) -> SRR_ADCU_FLR_OBJPos3_0x193FromOutData/1  "SRR_ADCU_FLR_OBJPos3_0x193FromOutData"
  SRR_ADCU_FLR_OBJPos3_0x193FromInData/1 -> SRR_ADCU_FLR_OBJPos3_0x193/1(SRR_ADCU_FLR_OBJPos3_0x193FromInData)  "SRR_ADCU_FLR_OBJPos3_0x193FromInData"
  SRR_ADCU_FLR_OBJPos4_0x194/1(SRR_ADCU_FLR_OBJPos4_0x194FromOutData) -> SRR_ADCU_FLR_OBJPos4_0x194FromOutData/1  "SRR_ADCU_FLR_OBJPos4_0x194FromOutData"
  SRR_ADCU_FLR_OBJPos4_0x194FromInData/1 -> SRR_ADCU_FLR_OBJPos4_0x194/1(SRR_ADCU_FLR_OBJPos4_0x194FromInData)  "SRR_ADCU_FLR_OBJPos4_0x194FromInData"
  SRR_ADCU_FLR_OBJPos5_0x195/1(SRR_ADCU_FLR_OBJPos5_0x195FromOutData) -> SRR_ADCU_FLR_OBJPos5_0x195FromOutData/1  "SRR_ADCU_FLR_OBJPos5_0x195FromOutData"
  SRR_ADCU_FLR_OBJPos5_0x195FromInData/1 -> SRR_ADCU_FLR_OBJPos5_0x195/1(SRR_ADCU_FLR_OBJPos5_0x195FromInData)  "SRR_ADCU_FLR_OBJPos5_0x195FromInData"
  SRR_ADCU_FLR_OBJPos6_0x196/1(SRR_ADCU_FLR_OBJPos6_0x196FromOutData) -> SRR_ADCU_FLR_OBJPos6_0x196FromOutData/1  "SRR_ADCU_FLR_OBJPos6_0x196FromOutData"
  SRR_ADCU_FLR_OBJPos6_0x196FromInData/1 -> SRR_ADCU_FLR_OBJPos6_0x196/1(SRR_ADCU_FLR_OBJPos6_0x196FromInData)  "SRR_ADCU_FLR_OBJPos6_0x196FromInData"
  SRR_ADCU_FLR_OBJPos7_0x197/1(SRR_ADCU_FLR_OBJPos7_0x197FromOutData) -> SRR_ADCU_FLR_OBJPos7_0x197FromOutData/1  "SRR_ADCU_FLR_OBJPos7_0x197FromOutData"
  SRR_ADCU_FLR_OBJPos7_0x197FromInData/1 -> SRR_ADCU_FLR_OBJPos7_0x197/1(SRR_ADCU_FLR_OBJPos7_0x197FromInData)  "SRR_ADCU_FLR_OBJPos7_0x197FromInData"
  SRR_ADCU_FLR_OBJPos8_0x198/1(SRR_ADCU_FLR_OBJPos8_0x198FromOutData) -> SRR_ADCU_FLR_OBJPos8_0x198FromOutData/1  "SRR_ADCU_FLR_OBJPos8_0x198FromOutData"
  SRR_ADCU_FLR_OBJPos8_0x198FromInData/1 -> SRR_ADCU_FLR_OBJPos8_0x198/1(SRR_ADCU_FLR_OBJPos8_0x198FromInData)  "SRR_ADCU_FLR_OBJPos8_0x198FromInData"
  SRR_ADCU_FLR_OBJPos9_0x199/1(SRR_ADCU_FLR_OBJPos9_0x199FromOutData) -> SRR_ADCU_FLR_OBJPos9_0x199FromOutData/1  "SRR_ADCU_FLR_OBJPos9_0x199FromOutData"
  SRR_ADCU_FLR_OBJPos9_0x199FromInData/1 -> SRR_ADCU_FLR_OBJPos9_0x199/1(SRR_ADCU_FLR_OBJPos9_0x199FromInData)  "SRR_ADCU_FLR_OBJPos9_0x199FromInData"
  SRR_ADCU_FRR_AssistSysSt_0x72/1(SRR_ADCU_FRR_AssistSysSt_0x72FromOutData) -> SRR_ADCU_FRR_AssistSysSt_0x72FromOutData/1  "SRR_ADCU_FRR_AssistSysSt_0x72FromOutData"
  SRR_ADCU_FRR_AssistSysSt_0x72FromInData/1 -> SRR_ADCU_FRR_AssistSysSt_0x72/1(SRR_ADCU_FRR_AssistSysSt_0x72FromInData)  "SRR_ADCU_FRR_AssistSysSt_0x72FromInData"
  SRR_ADCU_FRR_Freespace_1E6/1(SRR_ADCU_FRR_Freespace_1E6FromOutData) -> SRR_ADCU_FRR_Freespace_1E6FromOutData/1  "SRR_ADCU_FRR_Freespace_1E6FromOutData"
  SRR_ADCU_FRR_Freespace_1E6FromInData/1 -> SRR_ADCU_FRR_Freespace_1E6/1(SRR_ADCU_FRR_Freespace_1E6FromInData)  "SRR_ADCU_FRR_Freespace_1E6FromInData"
  SRR_ADCU_FRR_Freespace_1E7/1(SRR_ADCU_FRR_Freespace_1E7FromOutData) -> SRR_ADCU_FRR_Freespace_1E7FromOutData/1  "SRR_ADCU_FRR_Freespace_1E7FromOutData"
  SRR_ADCU_FRR_Freespace_1E7FromInData/1 -> SRR_ADCU_FRR_Freespace_1E7/1(SRR_ADCU_FRR_Freespace_1E7FromInData)  "SRR_ADCU_FRR_Freespace_1E7FromInData"
  SRR_ADCU_FRR_Freespace_1E8/1(SRR_ADCU_FRR_Freespace_1E8FromOutData) -> SRR_ADCU_FRR_Freespace_1E8FromOutData/1  "SRR_ADCU_FRR_Freespace_1E8FromOutData"
  SRR_ADCU_FRR_Freespace_1E8FromInData/1 -> SRR_ADCU_FRR_Freespace_1E8/1(SRR_ADCU_FRR_Freespace_1E8FromInData)  "SRR_ADCU_FRR_Freespace_1E8FromInData"
  SRR_ADCU_FRR_Freespace_1E9/1(SRR_ADCU_FRR_Freespace_1E9FromOutData) -> SRR_ADCU_FRR_Freespace_1E9FromOutData/1  "SRR_ADCU_FRR_Freespace_1E9FromOutData"
  SRR_ADCU_FRR_Freespace_1E9FromInData/1 -> SRR_ADCU_FRR_Freespace_1E9/1(SRR_ADCU_FRR_Freespace_1E9FromInData)  "SRR_ADCU_FRR_Freespace_1E9FromInData"
  SRR_ADCU_FRR_OBJPos10_0x1AC/1(SRR_ADCU_FRR_OBJPos10_0x1ACFromOutData) -> SRR_ADCU_FRR_OBJPos10_0x1ACFromOutData/1  "SRR_ADCU_FRR_OBJPos10_0x1ACFromOutData"
  SRR_ADCU_FRR_OBJPos10_0x1ACFromInData/1 -> SRR_ADCU_FRR_OBJPos10_0x1AC/1(SRR_ADCU_FRR_OBJPos10_0x1ACFromInData)  "SRR_ADCU_FRR_OBJPos10_0x1ACFromInData"
  SRR_ADCU_FRR_OBJPos11_0x1AD/1(SRR_ADCU_FRR_OBJPos11_0x1ADFromOutData) -> SRR_ADCU_FRR_OBJPos11_0x1ADFromOutData/1  "SRR_ADCU_FRR_OBJPos11_0x1ADFromOutData"
  SRR_ADCU_FRR_OBJPos11_0x1ADFromInData/1 -> SRR_ADCU_FRR_OBJPos11_0x1AD/1(SRR_ADCU_FRR_OBJPos11_0x1ADFromInData)  "SRR_ADCU_FRR_OBJPos11_0x1ADFromInData"
  SRR_ADCU_FRR_OBJPos12_0x1AE/1(SRR_ADCU_FRR_OBJPos12_0x1AEFromOutData) -> SRR_ADCU_FRR_OBJPos12_0x1AEFromOutData/1  "SRR_ADCU_FRR_OBJPos12_0x1AEFromOutData"
  SRR_ADCU_FRR_OBJPos12_0x1AEFromInData/1 -> SRR_ADCU_FRR_OBJPos12_0x1AE/1(SRR_ADCU_FRR_OBJPos12_0x1AEFromInData)  "SRR_ADCU_FRR_OBJPos12_0x1AEFromInData"
  SRR_ADCU_FRR_OBJPos13_0x1B0/1(SRR_ADCU_FRR_OBJPos13_0x1B0FromOutData) -> SRR_ADCU_FRR_OBJPos13_0x1B0FromOutData/1  "SRR_ADCU_FRR_OBJPos13_0x1B0FromOutData"
  SRR_ADCU_FRR_OBJPos13_0x1B0FromInData/1 -> SRR_ADCU_FRR_OBJPos13_0x1B0/1(SRR_ADCU_FRR_OBJPos13_0x1B0FromInData)  "SRR_ADCU_FRR_OBJPos13_0x1B0FromInData"
  SRR_ADCU_FRR_OBJPos14_0x1B1/1(SRR_ADCU_FRR_OBJPos14_0x1B1FromOutData) -> SRR_ADCU_FRR_OBJPos14_0x1B1FromOutData/1  "SRR_ADCU_FRR_OBJPos14_0x1B1FromOutData"
  SRR_ADCU_FRR_OBJPos14_0x1B1FromInData/1 -> SRR_ADCU_FRR_OBJPos14_0x1B1/1(SRR_ADCU_FRR_OBJPos14_0x1B1FromInData)  "SRR_ADCU_FRR_OBJPos14_0x1B1FromInData"
  SRR_ADCU_FRR_OBJPos15_0x1B2/1(SRR_ADCU_FRR_OBJPos15_0x1B2FromOutData) -> SRR_ADCU_FRR_OBJPos15_0x1B2FromOutData/1  "SRR_ADCU_FRR_OBJPos15_0x1B2FromOutData"
  SRR_ADCU_FRR_OBJPos15_0x1B2FromInData/1 -> SRR_ADCU_FRR_OBJPos15_0x1B2/1(SRR_ADCU_FRR_OBJPos15_0x1B2FromInData)  "SRR_ADCU_FRR_OBJPos15_0x1B2FromInData"
  SRR_ADCU_FRR_OBJPos16_0x1B3/1(SRR_ADCU_FRR_OBJPos16_0x1B3FromOutData) -> SRR_ADCU_FRR_OBJPos16_0x1B3FromOutData/1  "SRR_ADCU_FRR_OBJPos16_0x1B3FromOutData"
  SRR_ADCU_FRR_OBJPos16_0x1B3FromInData/1 -> SRR_ADCU_FRR_OBJPos16_0x1B3/1(SRR_ADCU_FRR_OBJPos16_0x1B3FromInData)  "SRR_ADCU_FRR_OBJPos16_0x1B3FromInData"
  SRR_ADCU_FRR_OBJPos1_0x1A3/1(SRR_ADCU_FRR_OBJPos1_0x1A3FromOutData) -> SRR_ADCU_FRR_OBJPos1_0x1A3FromOutData/1  "SRR_ADCU_FRR_OBJPos1_0x1A3FromOutData"
  SRR_ADCU_FRR_OBJPos1_0x1A3FromInData/1 -> SRR_ADCU_FRR_OBJPos1_0x1A3/1(SRR_ADCU_FRR_OBJPos1_0x1A3FromInData)  "SRR_ADCU_FRR_OBJPos1_0x1A3FromInData"
  SRR_ADCU_FRR_OBJPos2_0x1A4/1(SRR_ADCU_FRR_OBJPos2_0x1A4FromOutData) -> SRR_ADCU_FRR_OBJPos2_0x1A4FromOutData/1  "SRR_ADCU_FRR_OBJPos2_0x1A4FromOutData"
  SRR_ADCU_FRR_OBJPos2_0x1A4FromInData/1 -> SRR_ADCU_FRR_OBJPos2_0x1A4/1(SRR_ADCU_FRR_OBJPos2_0x1A4FromInData)  "SRR_ADCU_FRR_OBJPos2_0x1A4FromInData"
  SRR_ADCU_FRR_OBJPos3_0x1A5/1(SRR_ADCU_FRR_OBJPos3_0x1A5FromOutData) -> SRR_ADCU_FRR_OBJPos3_0x1A5FromOutData/1  "SRR_ADCU_FRR_OBJPos3_0x1A5FromOutData"
  SRR_ADCU_FRR_OBJPos3_0x1A5FromInData/1 -> SRR_ADCU_FRR_OBJPos3_0x1A5/1(SRR_ADCU_FRR_OBJPos3_0x1A5FromInData)  "SRR_ADCU_FRR_OBJPos3_0x1A5FromInData"
  SRR_ADCU_FRR_OBJPos4_0x1A6/1(SRR_ADCU_FRR_OBJPos4_0x1A6FromOutData) -> SRR_ADCU_FRR_OBJPos4_0x1A6FromOutData/1  "SRR_ADCU_FRR_OBJPos4_0x1A6FromOutData"
  SRR_ADCU_FRR_OBJPos4_0x1A6FromInData/1 -> SRR_ADCU_FRR_OBJPos4_0x1A6/1(SRR_ADCU_FRR_OBJPos4_0x1A6FromInData)  "SRR_ADCU_FRR_OBJPos4_0x1A6FromInData"
  SRR_ADCU_FRR_OBJPos5_0x1A7/1(SRR_ADCU_FRR_OBJPos5_0x1A7FromOutData) -> SRR_ADCU_FRR_OBJPos5_0x1A7FromOutData/1  "SRR_ADCU_FRR_OBJPos5_0x1A7FromOutData"
  SRR_ADCU_FRR_OBJPos5_0x1A7FromInData/1 -> SRR_ADCU_FRR_OBJPos5_0x1A7/1(SRR_ADCU_FRR_OBJPos5_0x1A7FromInData)  "SRR_ADCU_FRR_OBJPos5_0x1A7FromInData"
  SRR_ADCU_FRR_OBJPos6_0x1A8/1(SRR_ADCU_FRR_OBJPos6_0x1A8FromOutData) -> SRR_ADCU_FRR_OBJPos6_0x1A8FromOutData/1  "SRR_ADCU_FRR_OBJPos6_0x1A8FromOutData"
  SRR_ADCU_FRR_OBJPos6_0x1A8FromInData/1 -> SRR_ADCU_FRR_OBJPos6_0x1A8/1(SRR_ADCU_FRR_OBJPos6_0x1A8FromInData)  "SRR_ADCU_FRR_OBJPos6_0x1A8FromInData"
  SRR_ADCU_FRR_OBJPos7_0x1A9/1(SRR_ADCU_FRR_OBJPos7_0x1A9FromOutData) -> SRR_ADCU_FRR_OBJPos7_0x1A9FromOutData/1  "SRR_ADCU_FRR_OBJPos7_0x1A9FromOutData"
  SRR_ADCU_FRR_OBJPos7_0x1A9FromInData/1 -> SRR_ADCU_FRR_OBJPos7_0x1A9/1(SRR_ADCU_FRR_OBJPos7_0x1A9FromInData)  "SRR_ADCU_FRR_OBJPos7_0x1A9FromInData"
  SRR_ADCU_FRR_OBJPos8_0x1AA/1(SRR_ADCU_FRR_OBJPos8_0x1AAFromOutData) -> SRR_ADCU_FRR_OBJPos8_0x1AAFromOutData/1  "SRR_ADCU_FRR_OBJPos8_0x1AAFromOutData"
  SRR_ADCU_FRR_OBJPos8_0x1AAFromInData/1 -> SRR_ADCU_FRR_OBJPos8_0x1AA/1(SRR_ADCU_FRR_OBJPos8_0x1AAFromInData)  "SRR_ADCU_FRR_OBJPos8_0x1AAFromInData"
  SRR_ADCU_FRR_OBJPos9_0x1AB/1(SRR_ADCU_FRR_OBJPos9_0x1ABFromOutData) -> SRR_ADCU_FRR_OBJPos9_0x1ABFromOutData/1  "SRR_ADCU_FRR_OBJPos9_0x1ABFromOutData"
  SRR_ADCU_FRR_OBJPos9_0x1ABFromInData/1 -> SRR_ADCU_FRR_OBJPos9_0x1AB/1(SRR_ADCU_FRR_OBJPos9_0x1ABFromInData)  "SRR_ADCU_FRR_OBJPos9_0x1ABFromInData"
  SRR_ADCU_RLR_AssistSysSt_0x74/1(SRR_ADCU_RLR_AssistSysSt_0x74FromOutData) -> SRR_ADCU_RLR_AssistSysSt_0x74FromOutData/1  "SRR_ADCU_RLR_AssistSysSt_0x74FromOutData"
  SRR_ADCU_RLR_AssistSysSt_0x74FromInData/1 -> SRR_ADCU_RLR_AssistSysSt_0x74/1(SRR_ADCU_RLR_AssistSysSt_0x74FromInData)  "SRR_ADCU_RLR_AssistSysSt_0x74FromInData"
  SRR_ADCU_RLR_Freespace_0x1F1/1(SRR_ADCU_RLR_Freespace_0x1F1FromOutData) -> SRR_ADCU_RLR_Freespace_0x1F1FromOutData/1  "SRR_ADCU_RLR_Freespace_0x1F1FromOutData"
  SRR_ADCU_RLR_Freespace_0x1F1FromInData/1 -> SRR_ADCU_RLR_Freespace_0x1F1/1(SRR_ADCU_RLR_Freespace_0x1F1FromInData)  "SRR_ADCU_RLR_Freespace_0x1F1FromInData"
  SRR_ADCU_RLR_Freespace_0x1F2/1(SRR_ADCU_RLR_Freespace_0x1F2FromOutData) -> SRR_ADCU_RLR_Freespace_0x1F2FromOutData/1  "SRR_ADCU_RLR_Freespace_0x1F2FromOutData"
  SRR_ADCU_RLR_Freespace_0x1F2FromInData/1 -> SRR_ADCU_RLR_Freespace_0x1F2/1(SRR_ADCU_RLR_Freespace_0x1F2FromInData)  "SRR_ADCU_RLR_Freespace_0x1F2FromInData"
  SRR_ADCU_RLR_Freespace_0x1F3/1(SRR_ADCU_RLR_Freespace_0x1F3FromOutData) -> SRR_ADCU_RLR_Freespace_0x1F3FromOutData/1  "SRR_ADCU_RLR_Freespace_0x1F3FromOutData"
  SRR_ADCU_RLR_Freespace_0x1F3FromInData/1 -> SRR_ADCU_RLR_Freespace_0x1F3/1(SRR_ADCU_RLR_Freespace_0x1F3FromInData)  "SRR_ADCU_RLR_Freespace_0x1F3FromInData"
  SRR_ADCU_RLR_Freespace_0x1F4/1(SRR_ADCU_RLR_Freespace_0x1F4FromOutData) -> SRR_ADCU_RLR_Freespace_0x1F4FromOutData/1  "SRR_ADCU_RLR_Freespace_0x1F4FromOutData"
  SRR_ADCU_RLR_Freespace_0x1F4FromInData/1 -> SRR_ADCU_RLR_Freespace_0x1F4/1(SRR_ADCU_RLR_Freespace_0x1F4FromInData)  "SRR_ADCU_RLR_Freespace_0x1F4FromInData"
  SRR_ADCU_RLR_OBJPos10_0x1CD/1(SRR_ADCU_RLR_OBJPos10_0x1CDFromOutData) -> SRR_ADCU_RLR_OBJPos10_0x1CDFromOutData/1  "SRR_ADCU_RLR_OBJPos10_0x1CDFromOutData"
  SRR_ADCU_RLR_OBJPos10_0x1CDFromInData/1 -> SRR_ADCU_RLR_OBJPos10_0x1CD/1(SRR_ADCU_RLR_OBJPos10_0x1CDFromInData)  "SRR_ADCU_RLR_OBJPos10_0x1CDFromInData"
  SRR_ADCU_RLR_OBJPos11_0x1CE/1(SRR_ADCU_RLR_OBJPos11_0x1CEFromOutData) -> SRR_ADCU_RLR_OBJPos11_0x1CEFromOutData/1  "SRR_ADCU_RLR_OBJPos11_0x1CEFromOutData"
  SRR_ADCU_RLR_OBJPos11_0x1CEFromInData/1 -> SRR_ADCU_RLR_OBJPos11_0x1CE/1(SRR_ADCU_RLR_OBJPos11_0x1CEFromInData)  "SRR_ADCU_RLR_OBJPos11_0x1CEFromInData"
  SRR_ADCU_RLR_OBJPos12_0x1D1/1(SRR_ADCU_RLR_OBJPos12_0x1D1FromOutData) -> SRR_ADCU_RLR_OBJPos12_0x1D1FromOutData/1  "SRR_ADCU_RLR_OBJPos12_0x1D1FromOutData"
  SRR_ADCU_RLR_OBJPos12_0x1D1FromInData/1 -> SRR_ADCU_RLR_OBJPos12_0x1D1/1(SRR_ADCU_RLR_OBJPos12_0x1D1FromInData)  "SRR_ADCU_RLR_OBJPos12_0x1D1FromInData"
  SRR_ADCU_RLR_OBJPos13_0x1D2/1(SRR_ADCU_RLR_OBJPos13_0x1D2FromOutData) -> SRR_ADCU_RLR_OBJPos13_0x1D2FromOutData/1  "SRR_ADCU_RLR_OBJPos13_0x1D2FromOutData"
  SRR_ADCU_RLR_OBJPos13_0x1D2FromInData/1 -> SRR_ADCU_RLR_OBJPos13_0x1D2/1(SRR_ADCU_RLR_OBJPos13_0x1D2FromInData)  "SRR_ADCU_RLR_OBJPos13_0x1D2FromInData"
  SRR_ADCU_RLR_OBJPos14_0x1D3/1(SRR_ADCU_RLR_OBJPos14_0x1D3FromOutData) -> SRR_ADCU_RLR_OBJPos14_0x1D3FromOutData/1  "SRR_ADCU_RLR_OBJPos14_0x1D3FromOutData"
  SRR_ADCU_RLR_OBJPos14_0x1D3FromInData/1 -> SRR_ADCU_RLR_OBJPos14_0x1D3/1(SRR_ADCU_RLR_OBJPos14_0x1D3FromInData)  "SRR_ADCU_RLR_OBJPos14_0x1D3FromInData"
  SRR_ADCU_RLR_OBJPos15_0x1D4/1(SRR_ADCU_RLR_OBJPos15_0x1D4FromOutData) -> SRR_ADCU_RLR_OBJPos15_0x1D4FromOutData/1  "SRR_ADCU_RLR_OBJPos15_0x1D4FromOutData"
  SRR_ADCU_RLR_OBJPos15_0x1D4FromInData/1 -> SRR_ADCU_RLR_OBJPos15_0x1D4/1(SRR_ADCU_RLR_OBJPos15_0x1D4FromInData)  "SRR_ADCU_RLR_OBJPos15_0x1D4FromInData"
  SRR_ADCU_RLR_OBJPos16_0x1D5/1(SRR_ADCU_RLR_OBJPos16_0x1D5FromOutData) -> SRR_ADCU_RLR_OBJPos16_0x1D5FromOutData/1  "SRR_ADCU_RLR_OBJPos16_0x1D5FromOutData"
  SRR_ADCU_RLR_OBJPos16_0x1D5FromInData/1 -> SRR_ADCU_RLR_OBJPos16_0x1D5/1(SRR_ADCU_RLR_OBJPos16_0x1D5FromInData)  "SRR_ADCU_RLR_OBJPos16_0x1D5FromInData"
  SRR_ADCU_RLR_OBJPos1_0x1C4/1(SRR_ADCU_RLR_OBJPos1_0x1C4FromOutData) -> SRR_ADCU_RLR_OBJPos1_0x1C4FromOutData/1  "SRR_ADCU_RLR_OBJPos1_0x1C4FromOutData"
  SRR_ADCU_RLR_OBJPos1_0x1C4FromInData/1 -> SRR_ADCU_RLR_OBJPos1_0x1C4/1(SRR_ADCU_RLR_OBJPos1_0x1C4FromInData)  "SRR_ADCU_RLR_OBJPos1_0x1C4FromInData"
  SRR_ADCU_RLR_OBJPos2_0x1C5/1(SRR_ADCU_RLR_OBJPos2_0x1C5FromOutData) -> SRR_ADCU_RLR_OBJPos2_0x1C5FromOutData/1  "SRR_ADCU_RLR_OBJPos2_0x1C5FromOutData"
  SRR_ADCU_RLR_OBJPos2_0x1C5FromInData/1 -> SRR_ADCU_RLR_OBJPos2_0x1C5/1(SRR_ADCU_RLR_OBJPos2_0x1C5FromInData)  "SRR_ADCU_RLR_OBJPos2_0x1C5FromInData"
  SRR_ADCU_RLR_OBJPos3_0x1C6/1(SRR_ADCU_RLR_OBJPos3_0x1C6FromOutData) -> SRR_ADCU_RLR_OBJPos3_0x1C6FromOutData/1  "SRR_ADCU_RLR_OBJPos3_0x1C6FromOutData"
  SRR_ADCU_RLR_OBJPos3_0x1C6FromInData/1 -> SRR_ADCU_RLR_OBJPos3_0x1C6/1(SRR_ADCU_RLR_OBJPos3_0x1C6FromInData)  "SRR_ADCU_RLR_OBJPos3_0x1C6FromInData"
  SRR_ADCU_RLR_OBJPos4_0x1C7/1(SRR_ADCU_RLR_OBJPos4_0x1C7FromOutData) -> SRR_ADCU_RLR_OBJPos4_0x1C7FromOutData/1  "SRR_ADCU_RLR_OBJPos4_0x1C7FromOutData"
  SRR_ADCU_RLR_OBJPos4_0x1C7FromInData/1 -> SRR_ADCU_RLR_OBJPos4_0x1C7/1(SRR_ADCU_RLR_OBJPos4_0x1C7FromInData)  "SRR_ADCU_RLR_OBJPos4_0x1C7FromInData"
  SRR_ADCU_RLR_OBJPos5_0x1C8/1(SRR_ADCU_RLR_OBJPos5_0x1C8FromOutData) -> SRR_ADCU_RLR_OBJPos5_0x1C8FromOutData/1  "SRR_ADCU_RLR_OBJPos5_0x1C8FromOutData"
  SRR_ADCU_RLR_OBJPos5_0x1C8FromInData/1 -> SRR_ADCU_RLR_OBJPos5_0x1C8/1(SRR_ADCU_RLR_OBJPos5_0x1C8FromInData)  "SRR_ADCU_RLR_OBJPos5_0x1C8FromInData"
  SRR_ADCU_RLR_OBJPos6_0x1C9/1(SRR_ADCU_RLR_OBJPos6_0x1C9FromOutData) -> SRR_ADCU_RLR_OBJPos6_0x1C9FromOutData/1  "SRR_ADCU_RLR_OBJPos6_0x1C9FromOutData"
  SRR_ADCU_RLR_OBJPos6_0x1C9FromInData/1 -> SRR_ADCU_RLR_OBJPos6_0x1C9/1(SRR_ADCU_RLR_OBJPos6_0x1C9FromInData)  "SRR_ADCU_RLR_OBJPos6_0x1C9FromInData"
  SRR_ADCU_RLR_OBJPos7_0x1CA/1(SRR_ADCU_RLR_OBJPos7_0x1CAFromOutData) -> SRR_ADCU_RLR_OBJPos7_0x1CAFromOutData/1  "SRR_ADCU_RLR_OBJPos7_0x1CAFromOutData"
  SRR_ADCU_RLR_OBJPos7_0x1CAFromInData/1 -> SRR_ADCU_RLR_OBJPos7_0x1CA/1(SRR_ADCU_RLR_OBJPos7_0x1CAFromInData)  "SRR_ADCU_RLR_OBJPos7_0x1CAFromInData"
  SRR_ADCU_RLR_OBJPos8_0x1CB/1(SRR_ADCU_RLR_OBJPos8_0x1CBFromOutData) -> SRR_ADCU_RLR_OBJPos8_0x1CBFromOutData/1  "SRR_ADCU_RLR_OBJPos8_0x1CBFromOutData"
  SRR_ADCU_RLR_OBJPos8_0x1CBFromInData/1 -> SRR_ADCU_RLR_OBJPos8_0x1CB/1(SRR_ADCU_RLR_OBJPos8_0x1CBFromInData)  "SRR_ADCU_RLR_OBJPos8_0x1CBFromInData"
  SRR_ADCU_RLR_OBJPos9_0x1CC/1(SRR_ADCU_RLR_OBJPos9_0x1CCFromOutData) -> SRR_ADCU_RLR_OBJPos9_0x1CCFromOutData/1  "SRR_ADCU_RLR_OBJPos9_0x1CCFromOutData"
  SRR_ADCU_RLR_OBJPos9_0x1CCFromInData/1 -> SRR_ADCU_RLR_OBJPos9_0x1CC/1(SRR_ADCU_RLR_OBJPos9_0x1CCFromInData)  "SRR_ADCU_RLR_OBJPos9_0x1CCFromInData"
  SRR_ADCU_RRR_AssistSysSt_0x73/1(SRR_ADCU_RRR_AssistSysSt_0x73FromOutData) -> SRR_ADCU_RRR_AssistSysSt_0x73FromOutData/1  "SRR_ADCU_RRR_AssistSysSt_0x73FromOutData"
  SRR_ADCU_RRR_AssistSysSt_0x73FromInData/1 -> SRR_ADCU_RRR_AssistSysSt_0x73/1(SRR_ADCU_RRR_AssistSysSt_0x73FromInData)  "SRR_ADCU_RRR_AssistSysSt_0x73FromInData"
  SRR_ADCU_RRR_Freespace_0x1EB/1(SRR_ADCU_RRR_Freespace_0x1EBFromOutData) -> SRR_ADCU_RRR_Freespace_0x1EBFromOutData/1  "SRR_ADCU_RRR_Freespace_0x1EBFromOutData"
  SRR_ADCU_RRR_Freespace_0x1EBFromInData/1 -> SRR_ADCU_RRR_Freespace_0x1EB/1(SRR_ADCU_RRR_Freespace_0x1EBFromInData)  "SRR_ADCU_RRR_Freespace_0x1EBFromInData"
  SRR_ADCU_RRR_Freespace_0x1EC/1(SRR_ADCU_RRR_Freespace_0x1ECFromOutData) -> SRR_ADCU_RRR_Freespace_0x1ECFromOutData/1  "SRR_ADCU_RRR_Freespace_0x1ECFromOutData"
  SRR_ADCU_RRR_Freespace_0x1ECFromInData/1 -> SRR_ADCU_RRR_Freespace_0x1EC/1(SRR_ADCU_RRR_Freespace_0x1ECFromInData)  "SRR_ADCU_RRR_Freespace_0x1ECFromInData"
  SRR_ADCU_RRR_Freespace_0x1ED/1(SRR_ADCU_RRR_Freespace_0x1EDFromOutData) -> SRR_ADCU_RRR_Freespace_0x1EDFromOutData/1  "SRR_ADCU_RRR_Freespace_0x1EDFromOutData"
  SRR_ADCU_RRR_Freespace_0x1EDFromInData/1 -> SRR_ADCU_RRR_Freespace_0x1ED/1(SRR_ADCU_RRR_Freespace_0x1EDFromInData)  "SRR_ADCU_RRR_Freespace_0x1EDFromInData"
  SRR_ADCU_RRR_Freespace_0x1EE/1(SRR_ADCU_RRR_Freespace_0x1EEFromOutData) -> SRR_ADCU_RRR_Freespace_0x1EEFromOutData/1  "SRR_ADCU_RRR_Freespace_0x1EEFromOutData"
  SRR_ADCU_RRR_Freespace_0x1EEFromInData/1 -> SRR_ADCU_RRR_Freespace_0x1EE/1(SRR_ADCU_RRR_Freespace_0x1EEFromInData)  "SRR_ADCU_RRR_Freespace_0x1EEFromInData"
  SRR_ADCU_RRR_OBJPos10_0x1BD/1(SRR_ADCU_RRR_OBJPos10_0x1BDFromOutData) -> SRR_ADCU_RRR_OBJPos10_0x1BDFromOutData/1  "SRR_ADCU_RRR_OBJPos10_0x1BDFromOutData"
  SRR_ADCU_RRR_OBJPos10_0x1BDFromInData/1 -> SRR_ADCU_RRR_OBJPos10_0x1BD/1(SRR_ADCU_RRR_OBJPos10_0x1BDFromInData)  "SRR_ADCU_RRR_OBJPos10_0x1BDFromInData"
  SRR_ADCU_RRR_OBJPos11_0x1BE/1(SRR_ADCU_RRR_OBJPos11_0x1BEFromOutData) -> SRR_ADCU_RRR_OBJPos11_0x1BEFromOutData/1  "SRR_ADCU_RRR_OBJPos11_0x1BEFromOutData"
  SRR_ADCU_RRR_OBJPos11_0x1BEFromInData/1 -> SRR_ADCU_RRR_OBJPos11_0x1BE/1(SRR_ADCU_RRR_OBJPos11_0x1BEFromInData)  "SRR_ADCU_RRR_OBJPos11_0x1BEFromInData"
  SRR_ADCU_RRR_OBJPos12_0x1BF/1(SRR_ADCU_RRR_OBJPos12_0x1BFFromOutData) -> SRR_ADCU_RRR_OBJPos12_0x1BFFromOutData/1  "SRR_ADCU_RRR_OBJPos12_0x1BFFromOutData"
  SRR_ADCU_RRR_OBJPos12_0x1BFFromInData/1 -> SRR_ADCU_RRR_OBJPos12_0x1BF/1(SRR_ADCU_RRR_OBJPos12_0x1BFFromInData)  "SRR_ADCU_RRR_OBJPos12_0x1BFFromInData"
  SRR_ADCU_RRR_OBJPos13_0x1C0/1(SRR_ADCU_RRR_OBJPos13_0x1C0FromOutData) -> SRR_ADCU_RRR_OBJPos13_0x1C0FromOutData/1  "SRR_ADCU_RRR_OBJPos13_0x1C0FromOutData"
  SRR_ADCU_RRR_OBJPos13_0x1C0FromInData/1 -> SRR_ADCU_RRR_OBJPos13_0x1C0/1(SRR_ADCU_RRR_OBJPos13_0x1C0FromInData)  "SRR_ADCU_RRR_OBJPos13_0x1C0FromInData"
  SRR_ADCU_RRR_OBJPos14_0x1C1/1(SRR_ADCU_RRR_OBJPos14_0x1C1FromOutData) -> SRR_ADCU_RRR_OBJPos14_0x1C1FromOutData/1  "SRR_ADCU_RRR_OBJPos14_0x1C1FromOutData"
  SRR_ADCU_RRR_OBJPos14_0x1C1FromInData/1 -> SRR_ADCU_RRR_OBJPos14_0x1C1/1(SRR_ADCU_RRR_OBJPos14_0x1C1FromInData)  "SRR_ADCU_RRR_OBJPos14_0x1C1FromInData"
  SRR_ADCU_RRR_OBJPos15_0x1C2/1(SRR_ADCU_RRR_OBJPos15_0x1C2FromOutData) -> SRR_ADCU_RRR_OBJPos15_0x1C2FromOutData/1  "SRR_ADCU_RRR_OBJPos15_0x1C2FromOutData"
  SRR_ADCU_RRR_OBJPos15_0x1C2FromInData/1 -> SRR_ADCU_RRR_OBJPos15_0x1C2/1(SRR_ADCU_RRR_OBJPos15_0x1C2FromInData)  "SRR_ADCU_RRR_OBJPos15_0x1C2FromInData"
  SRR_ADCU_RRR_OBJPos16_0x1C3/1(SRR_ADCU_RRR_OBJPos16_0x1C3FromOutData) -> SRR_ADCU_RRR_OBJPos16_0x1C3FromOutData/1  "SRR_ADCU_RRR_OBJPos16_0x1C3FromOutData"
  SRR_ADCU_RRR_OBJPos16_0x1C3FromInData/1 -> SRR_ADCU_RRR_OBJPos16_0x1C3/1(SRR_ADCU_RRR_OBJPos16_0x1C3FromInData)  "SRR_ADCU_RRR_OBJPos16_0x1C3FromInData"
  SRR_ADCU_RRR_OBJPos1_0x1B4/1(SRR_ADCU_RRR_OBJPos1_0x1B4FromOutData) -> SRR_ADCU_RRR_OBJPos1_0x1B4FromOutData/1  "SRR_ADCU_RRR_OBJPos1_0x1B4FromOutData"
  SRR_ADCU_RRR_OBJPos1_0x1B4FromInData/1 -> SRR_ADCU_RRR_OBJPos1_0x1B4/1(SRR_ADCU_RRR_OBJPos1_0x1B4FromInData)  "SRR_ADCU_RRR_OBJPos1_0x1B4FromInData"
  SRR_ADCU_RRR_OBJPos2_0x1B5/1(SRR_ADCU_RRR_OBJPos2_0x1B5FromOutData) -> SRR_ADCU_RRR_OBJPos2_0x1B5FromOutData/1  "SRR_ADCU_RRR_OBJPos2_0x1B5FromOutData"
  SRR_ADCU_RRR_OBJPos2_0x1B5FromInData/1 -> SRR_ADCU_RRR_OBJPos2_0x1B5/1(SRR_ADCU_RRR_OBJPos2_0x1B5FromInData)  "SRR_ADCU_RRR_OBJPos2_0x1B5FromInData"
  SRR_ADCU_RRR_OBJPos3_0x1B6/1(SRR_ADCU_RRR_OBJPos3_0x1B6FromOutData) -> SRR_ADCU_RRR_OBJPos3_0x1B6FromOutData/1  "SRR_ADCU_RRR_OBJPos3_0x1B6FromOutData"
  SRR_ADCU_RRR_OBJPos3_0x1B6FromInData/1 -> SRR_ADCU_RRR_OBJPos3_0x1B6/1(SRR_ADCU_RRR_OBJPos3_0x1B6FromInData)  "SRR_ADCU_RRR_OBJPos3_0x1B6FromInData"
  SRR_ADCU_RRR_OBJPos4_0x1B7/1(SRR_ADCU_RRR_OBJPos4_0x1B7FromOutData) -> SRR_ADCU_RRR_OBJPos4_0x1B7FromOutData/1  "SRR_ADCU_RRR_OBJPos4_0x1B7FromOutData"
  SRR_ADCU_RRR_OBJPos4_0x1B7FromInData/1 -> SRR_ADCU_RRR_OBJPos4_0x1B7/1(SRR_ADCU_RRR_OBJPos4_0x1B7FromInData)  "SRR_ADCU_RRR_OBJPos4_0x1B7FromInData"
  SRR_ADCU_RRR_OBJPos5_0x1B8/1(SRR_ADCU_RRR_OBJPos5_0x1B8FromOutData) -> SRR_ADCU_RRR_OBJPos5_0x1B8FromOutData/1  "SRR_ADCU_RRR_OBJPos5_0x1B8FromOutData"
  SRR_ADCU_RRR_OBJPos5_0x1B8FromInData/1 -> SRR_ADCU_RRR_OBJPos5_0x1B8/1(SRR_ADCU_RRR_OBJPos5_0x1B8FromInData)  "SRR_ADCU_RRR_OBJPos5_0x1B8FromInData"
  SRR_ADCU_RRR_OBJPos6_0x1B9/1(SRR_ADCU_RRR_OBJPos6_0x1B9FromOutData) -> SRR_ADCU_RRR_OBJPos6_0x1B9FromOutData/1  "SRR_ADCU_RRR_OBJPos6_0x1B9FromOutData"
  SRR_ADCU_RRR_OBJPos6_0x1B9FromInData/1 -> SRR_ADCU_RRR_OBJPos6_0x1B9/1(SRR_ADCU_RRR_OBJPos6_0x1B9FromInData)  "SRR_ADCU_RRR_OBJPos6_0x1B9FromInData"
  SRR_ADCU_RRR_OBJPos7_0x1BA/1(SRR_ADCU_RRR_OBJPos7_0x1BAFromOutData) -> SRR_ADCU_RRR_OBJPos7_0x1BAFromOutData/1  "SRR_ADCU_RRR_OBJPos7_0x1BAFromOutData"
  SRR_ADCU_RRR_OBJPos7_0x1BAFromInData/1 -> SRR_ADCU_RRR_OBJPos7_0x1BA/1(SRR_ADCU_RRR_OBJPos7_0x1BAFromInData)  "SRR_ADCU_RRR_OBJPos7_0x1BAFromInData"
  SRR_ADCU_RRR_OBJPos8_0x1BB/1(SRR_ADCU_RRR_OBJPos8_0x1BBFromOutData) -> SRR_ADCU_RRR_OBJPos8_0x1BBFromOutData/1  "SRR_ADCU_RRR_OBJPos8_0x1BBFromOutData"
  SRR_ADCU_RRR_OBJPos8_0x1BBFromInData/1 -> SRR_ADCU_RRR_OBJPos8_0x1BB/1(SRR_ADCU_RRR_OBJPos8_0x1BBFromInData)  "SRR_ADCU_RRR_OBJPos8_0x1BBFromInData"
  SRR_ADCU_RRR_OBJPos9_0x1BC/1(SRR_ADCU_RRR_OBJPos9_0x1BCFromOutData) -> SRR_ADCU_RRR_OBJPos9_0x1BCFromOutData/1  "SRR_ADCU_RRR_OBJPos9_0x1BCFromOutData"
  SRR_ADCU_RRR_OBJPos9_0x1BCFromInData/1 -> SRR_ADCU_RRR_OBJPos9_0x1BC/1(SRR_ADCU_RRR_OBJPos9_0x1BCFromInData)  "SRR_ADCU_RRR_OBJPos9_0x1BCFromInData"
